simulink model "AutomatedValetParking"  (R2026a)
settings: Solver=VariableStepAuto  StopTime=inf  FixedStep=1e-3
PreLoadFcn:
  | costmap = VorlageCostmapErstellen();
  | routeData= load('routePlanSL.mat');
  | routePlan= routeData.routePlan;
  | startPose = routePlan.StartPose(1, :);
  | centerToFront = 1.4;
  | centerToRear = 1.4;
  | helperCreateBus;
StopFcn:
  | clear helperSLVisualizePath
values from neighbouring files (symbols this model uses):
  lr = vehDims.RearOverhang  + (vehDims.Wheelbase / 2)    [Initialisierung.m]
undefined symbols (not defined in the file or in its folder): DiscIntNeverNeededParam
libraries: drivingvehiclecontroller x2, drivinglib x2, simulink_extras x2, autolibshared x1
CloseFcn:
  | clear plannerConfigBus ...
  | speedConfigBus ...
  | startPose ...
  | costmap ...
  | routeData ...
  | routePlan ...
  | centerToFront ...
  | centerToRear;
settings Model: Creator=The MathWorks, Inc.  LastModifiedBy=moritzhumberg
settings SolverCC: DecoupledContinuousIntegration=on  MinimalZcImpactIntegration=on
settings DebuggingCC: PregeneratedLibrarySubsystemCodeDiagnostic=none
settings RTWCC: GenCodeOnly=on  PackageGeneratedCodeAndArtifacts=on

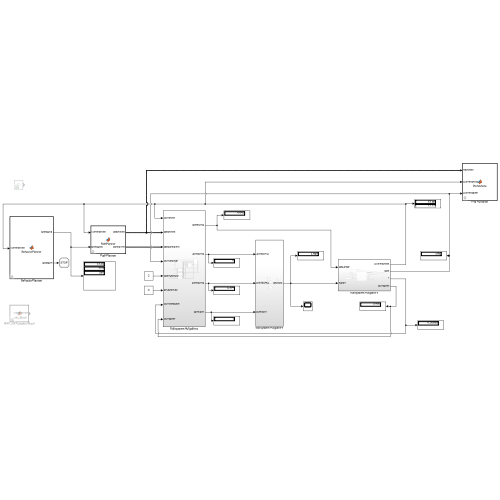
[thumbnail: Simulink's stored preview of the top-level diagram]
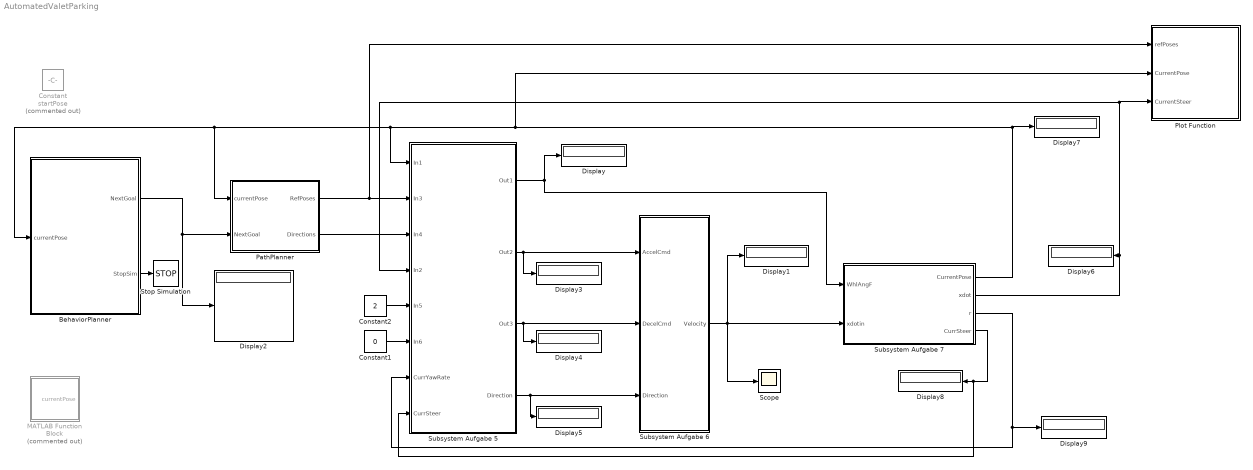
== system AutomatedValetParking ==
  BehaviorPlanner : MATLAB Function  TreatAsAtomicUnit=on  mask{routePlan=routePlan}
      mask init:
      | routePlanStruct = table2struct(routePlan);
  Constant : Constant  Commented=on  Value=startPose
  Constant1 : Constant  Value=0
  Constant2 : Constant  Value=2
  Display{,1..9} (10 alike) : Display
  MATLAB Function Block : MATLAB Function  Commented=on  TreatAsAtomicUnit=on
  PathPlanner : MATLAB Function  TreatAsAtomicUnit=on  mask{costmap=costmap}
      mask init:
      | varagout        = helperSLCreateUtilityStruct(costmap);
      |       vehicleDimsStruct = varagout{1};
      |       costmapStruct   = varagout{2};
  Plot Function : MATLAB Function  TreatAsAtomicUnit=on  mask{Costmap=costmap}
      mask init:
      | varagout        = helperSLCreateUtilityStruct(Costmap);
      |     vehicleDimsStruct = varagout{1};
      |     costmapStruct   = varagout{2};
  Scope : Scope
      settings: ActiveDisplayYMinimum=-1  ActiveDisplayYMaximum=1
  Stop Simulation : Stop
  Subsystem Aufgabe 5 : Subsystem
  Subsystem Aufgabe 6 : Subsystem
  Subsystem Aufgabe 7 : Subsystem
  wires:
  BehaviorPlanner/1(NextGoal) -> Display2/1, PathPlanner/2(NextGoal)
  PathPlanner/2(Directions) -> Subsystem Aufgabe 5/3(In4)
  PathPlanner/1(RefPoses) -> Plot Function/1(refPoses), Subsystem Aufgabe 5/2(In3)
  Constant2/1 -> Subsystem Aufgabe 5/5(In5)
  Subsystem Aufgabe 5/1(Out1) -> Subsystem Aufgabe 7/1(WhlAngF), Display/1
  Subsystem Aufgabe 6/1(Velocity) -> Scope/1, Subsystem Aufgabe 7/2(xdotin), Display1/1
  Subsystem Aufgabe 5/4(Direction) -> Display5/1, Subsystem Aufgabe 6/3(Direction)
  Subsystem Aufgabe 5/2(Out2) -> Display3/1, Subsystem Aufgabe 6/1(AccelCmd)
  Subsystem Aufgabe 5/3(Out3) -> Display4/1, Subsystem Aufgabe 6/2(DecelCmd)
  Subsystem Aufgabe 7/1(CurrentPose) -> Plot Function/2(CurrentPose), BehaviorPlanner/1(currentPose), PathPlanner/1(currentPose), Subsystem Aufgabe 5/1(In1), Display7/1
  Subsystem Aufgabe 7/2(xdot) -> Display6/1, Subsystem Aufgabe 5/4(In2), Plot Function/3(CurrentSteer)
  Subsystem Aufgabe 7/4(CurrSteer) -> Subsystem Aufgabe 5/8(CurrSteer), Display8/1
  Subsystem Aufgabe 7/3(r) -> Subsystem Aufgabe 5/7(CurrYawRate), Display9/1
  Constant1/1 -> Subsystem Aufgabe 5/6(In6)
  BehaviorPlanner/2(StopSim) -> Stop Simulation/1

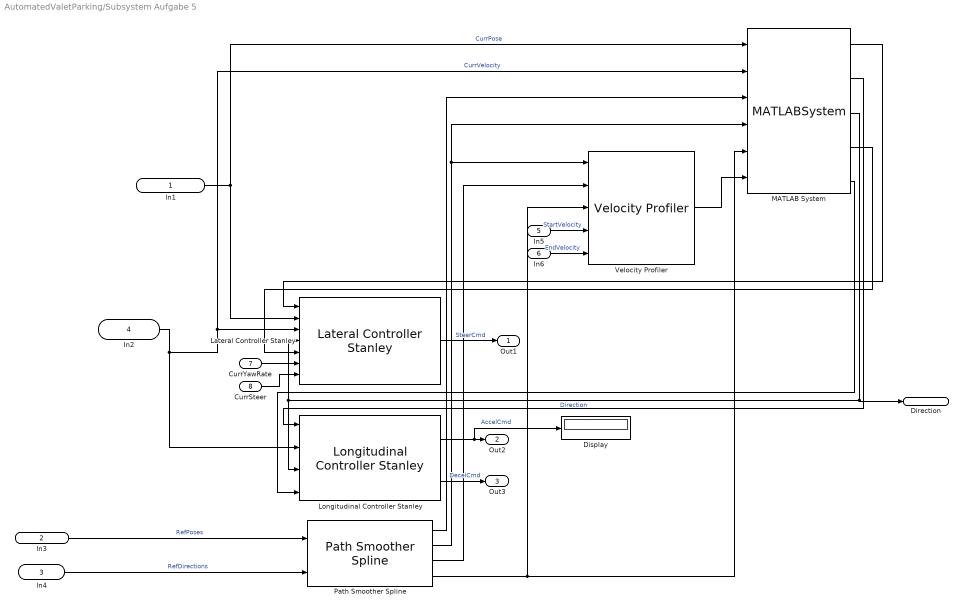
== system AutomatedValetParking/Subsystem Aufgabe 5 ==
  In1 : Inport
  In3 : Inport  Port=2
  In4 : Inport  Port=3
  In2 : Inport  Port=4
  In5 : Inport  Port=5
  In6 : Inport  Port=6
  CurrYawRate : Inport  Port=7
  CurrSteer : Inport  Port=8
  Display : Display
  Lateral Controller Stanley : drivingvehiclecontroller/Lateral Controller Stanley  ModelType=Dynamic bicycle model  PositionGainF=2.5  PositionGainR=2.5  YawRateGain=0.2  DelayGain=0.2  VehicleMass=1575  Lf=1.2  Lr=1.6  TireStiffness=19000  Wheelbase=2.8  MaxSteeringAngle=35
  Longitudinal Controller Stanley : drivingvehiclecontroller/Longitudinal Controller Stanley  Kp=2.5  Ki=1  SampleTime=0.1  MaxAcceleration=2  MaxDeceleration=4
  MATLAB System : MATLABSystem  System=HelperPathAnalyzer  Wheelbase=2.8  HasResetOutput=on  SimulateUsing=Interpreted execution
      mask Type: HelperPathAnalyzer
  Path Smoother Spline : drivinglib/Path Smoother Spline  NumSmoothPoses=100  MinSeparation=1e-3  SampleTime=0.1  ShowOptionalOutports=on  SimulateUsing=Interpreted execution
  Velocity Profiler : drivinglib/Velocity Profiler  MaxLongitudinalAccel=2  MaxLongitudinalDecel=4  MaxSpeed=10  MaxLongitudinalJerk=1  MaxLateralAccel=2  ShowOptionalOutport=off  SampleTime=-1  SimulateUsing=Code generation
  Out1 : Outport
  Out2 : Outport  Port=2
  Out3 : Outport  Port=3
  Direction : Outport  Port=4
  wires:
  In1/1 -> MATLAB System/1, Lateral Controller Stanley/2  "CurrPose"
  In2/1 -> Longitudinal Controller Stanley/2, MATLAB System/2, Lateral Controller Stanley/3  "CurrVelocity"
  In3/1 -> Path Smoother Spline/1  "RefPoses"
  Lateral Controller Stanley/1 -> Out1/1  "SteerCmd"
  Longitudinal Controller Stanley/1 -> Display/1, Out2/1  "AccelCmd"
  Longitudinal Controller Stanley/2 -> Out3/1  "DecelCmd"
  In5/1 -> Velocity Profiler/4  "StartVelocity"
  In6/1 -> Velocity Profiler/5  "EndVelocity"
  In4/1 -> Path Smoother Spline/2  "RefDirections"
  MATLAB System/3 -> Direction/1, Lateral Controller Stanley/4, Longitudinal Controller Stanley/3  "Direction"
  MATLAB System/1 -> Lateral Controller Stanley/1
  MATLAB System/2 -> Longitudinal Controller Stanley/1
  MATLAB System/5 -> Longitudinal Controller Stanley/4
  Path Smoother Spline/4 -> MATLAB System/5, Velocity Profiler/3
  Velocity Profiler/1 -> MATLAB System/6
  Path Smoother Spline/3 -> Velocity Profiler/2
  Path Smoother Spline/2 -> MATLAB System/4, Velocity Profiler/1
  Path Smoother Spline/1 -> MATLAB System/3
  MATLAB System/4 -> Lateral Controller Stanley/5
  CurrYawRate/1 -> Lateral Controller Stanley/6
  CurrSteer/1 -> Lateral Controller Stanley/7

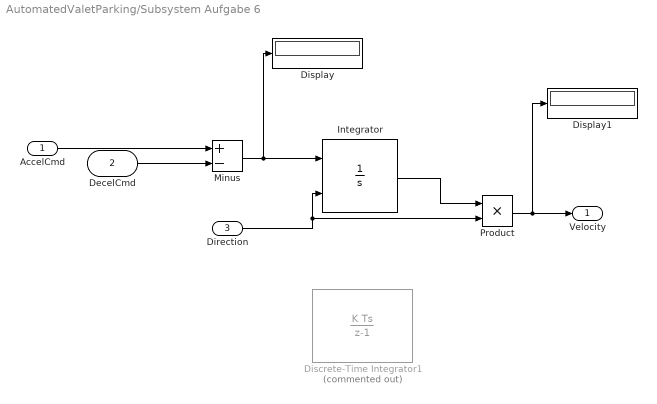
== system AutomatedValetParking/Subsystem Aufgabe 6 ==
  AccelCmd : Inport
  DecelCmd : Inport  Port=2
  Direction : Inport  Port=3
  Discrete-Time Integrator1 : DiscreteIntegrator  Commented=on  ExternalReset=either  InitialCondition=2  SampleTime=0.1  LimitOutput=on  LowerSaturationLimit=0  ICPrevOutput=DiscIntNeverNeededParam  ICPrevScaledInput=DiscIntNeverNeededParam
  Display : Display
  Display1 : Display
  Integrator : Integrator  ExternalReset=either  LimitOutput=on  LowerSaturationLimit=0
  Minus : Sum  Inputs=+-
  Product : Product
  Velocity : Outport
  wires:
  Minus/1 -> Integrator/1, Display/1
  DecelCmd/1 -> Minus/2
  AccelCmd/1 -> Minus/1
  Product/1 -> Velocity/1, Display1/1
  Direction/1 -> Integrator/2, Product/2
  Integrator/1 -> Product/1

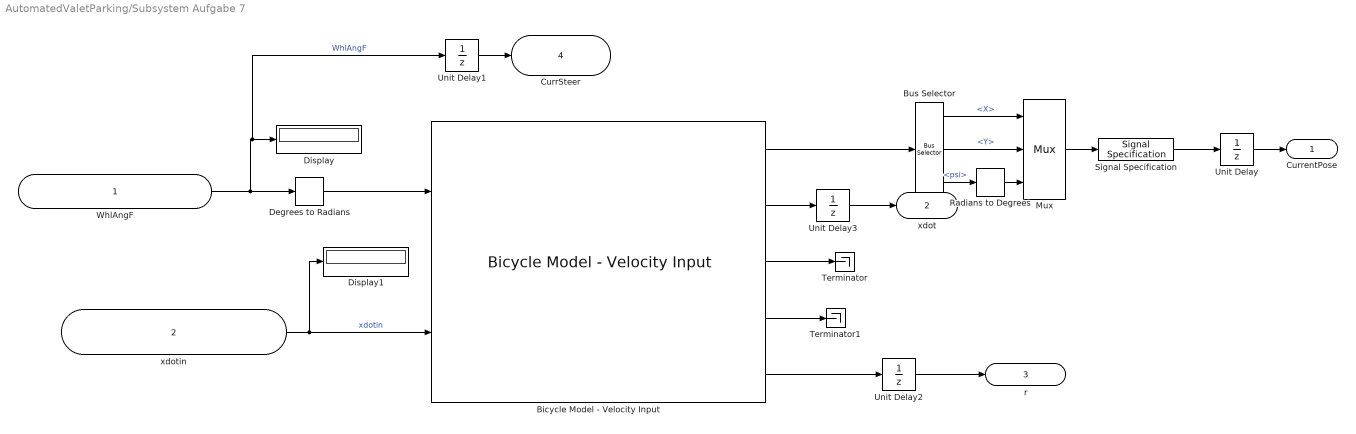
== system AutomatedValetParking/Subsystem Aufgabe 7 ==
  WhlAngF : Inport
  xdotin : Inport  Port=2
  Bicycle Model - Velocity Input : autolibshared/Bicycle Model - Velocity Input  trackMode=Single (bicycle)  inputMode=External longitudinal velocity  frontSteerMode=on  rearSteerMode=off  windMode=off  muMode=off  extFMode=off  extMMode=off  aMode=3  NF=2  NR=2  m=2000  a=lf  b=lr  h=0.35  X_o=startPose(1)  xdot_o=0  CalphaMode=Constant  sigmaMode=on  w=[1.4,1.4]  Cy_f=12e3  Cy_r=11e3  sigma_f=.1  sigma_r=.1  alpha_f_brk=[-.1 .1]  Cy_f_data=[-9e3 9e3]  alpha_r_brk=[-.1 .1]  Cy_r_data=[-9e3 9e3]  Y_o=startPose(2)  ydot_o=0  Izz=4000  psi_o=startPose(3)  r_o=0  Af=2  Cd=.3  Cl=.1  Cpm=.1  beta_w=[0 0.01:0.01:0.3]  Cs=[0 0.01:0.01:0.3]  Cym=[0 1e-6:0.01:0.3]  Pabs=101325  Tair=273  g=9.81  mu=1  xdot_tol=.01  Fznom=5000  Fxtire_sat=1e6  Fytire_sat=1e6  longOff=0  latOff=0  vertOff=0
      settings: LibrarySourceBlock=drivingscenarioandsensors/Bicycle Model - Velocity Input
  Bus Selector : BusSelector  OutputSignals=InertFrm.Cg.Disp.X,InertFrm.Cg.Disp.Y,InertFrm.Cg.Ang.psi
  Degrees to Radians : simulink_extras/Transformations/Degrees to Radians
  Display : Display
  Display1 : Display
  Mux : Mux  Inputs=3
  Radians to Degrees : simulink_extras/Transformations/Radians to Degrees
  Signal Specification : SignalSpecification  Dimensions=[1 3]
  Terminator : Terminator
  Terminator1 : Terminator
  Unit Delay : UnitDelay  InitialCondition=startPose  SampleTime=0.1
  Unit Delay1 : UnitDelay  SampleTime=-1
  Unit Delay2 : UnitDelay  SampleTime=-1
  Unit Delay3 : UnitDelay  SampleTime=-1
  CurrentPose : Outport
  xdot : Outport  Port=2
  r : Outport  Port=3
  CurrSteer : Outport  Port=4
  wires:
  Bicycle Model - Velocity Input/5 -> Unit Delay2/1
  Bicycle Model - Velocity Input/2 -> Unit Delay3/1
  WhlAngF/1 -> Unit Delay1/1, Display/1, Degrees to Radians/1  "WhlAngF"
  xdotin/1 -> Display1/1, Bicycle Model - Velocity Input/2  "xdotin"
  Degrees to Radians/1 -> Bicycle Model - Velocity Input/1
  Bicycle Model - Velocity Input/1 -> Bus Selector/1
  Bus Selector/1 -> Mux/1  "<X>"
  Bus Selector/2 -> Mux/2  "<Y>"
  Bus Selector/3 -> Radians to Degrees/1  "<psi>"
  Mux/1 -> Signal Specification/1
  Unit Delay1/1 -> CurrSteer/1
  Bicycle Model - Velocity Input/3 -> Terminator/1
  Bicycle Model - Velocity Input/4 -> Terminator1/1
  Unit Delay/1 -> CurrentPose/1
  Signal Specification/1 -> Unit Delay/1
  Unit Delay2/1 -> r/1
  Unit Delay3/1 -> xdot/1
  Radians to Degrees/1 -> Mux/3

== matlab function AutomatedValetParking/BehaviorPlanner ==
  settings: updateMethod=DISCRETE  sampleTime=0.1
  data: routePlanStruct parameter; NextGoal output size=1 3; currentPose input size=1 3; StopSim output
%% BehaviorPlanner
% Dieser Block soll aus dem routePlan die entsprechende Zielpose sowie 
% Geschwindigkeiten entnehmen und an dem motionPlaning Block
% weitergeben. Weiterhin soll der Block die Einstellung für den 
% RRT*-Algorithmus entsprechend der aktuellen Fahrsituation ermittlen und
% dem PathPlanner übergeben.
% Schließlich soll der Block nach dem Erreichen der finalen Zielpose die
% Simulation beenden.

% ------------------------------------------------------------------------------------------------------------
function [NextGoal, StopSim] = BehaviorPlanner(routePlanStruct, currentPose)

StopSim = false;
persistent GoalIndex;

if isempty(GoalIndex)
GoalIndex = 1; % Startwert
end

numGoals = length(routePlanStruct);

NextGoal = routePlanStruct(GoalIndex).EndPose;

dist = norm(currentPose(1:2) - NextGoal(1:2));

Toleranz = 0.8;




%% Aufgabe 3
% Nach der Definition der Ein- und Ausgänge der Function muss die Maske des
% Matlab Function Blocks definiert werden. Eine Besonderheit besteht darin,
% dass der routePlan aus Matlab geladen wird. 
% Aus diesem Grund ist dies kein klassischer Eingang vom Matlab 
% Function Block. 
% Unter Rechtsklick auf dem Matlab Function Block > Masks > Edit Mask...
% ist Parameters & Dialog zu finden. Dort können die Parameter definiert
% werden, die beim Doppelklick auf den Matlab Function Block definiert
% werden sollen.
% Unter dem Punkt Code lässt sich eine Intialisierungs Function
% definieren. Dieser Code wird benötigt um den routePlan in das Format
% "struct" zu konvertieren. Dies hat den Grund, dass Matlab Function Blöcke
% das Format "table" nicht unterstützen. Aus diesem Grund ist im Mask
% Editor unter Code über den Befehl 'S = table2struct(T)' eine Konvertierung
% des routePlans in ein Struct nötig. Ein Struct ist ein Datenformat, der
% aus einem großen "Container" besteht, in dem mehrere Werte eingegliedert
% sind. So lässt sich eine geordnetere Datenstruktur bilden.
% Weitere Erläuterungen zur Mask befinden sich unter Kapitel 5.3 in den
% Praktikumsunterlagen Aufgabenstellung.

% -

% Wenn nur eine erste Zielpose ausgegeben werden soll, reicht die
% Implementierung des GoalIndexes und der einfache
% Befehl x = routePlanStruct(Index).EndPose
%                  |           |        |
%           Variablenname  Zeilennr.  Spalte
% Der GoalIndex ist in dieser Aufgabe nur eine Konstante, da lediglich die 
% erste Zielpose aufgerufen werden soll. 
% In den aufbauenden Aufgaben wird dies aber eine laufende Nummer, die
% nacheinander alle Zielposen aus dem dem RoutePlan aufruft.
% Dieser Schritt wird in folgenden Aufgaben aber in requestManeuver.m
% ausgelagert, da dies bei komplexeren Anwendungen Vorteile hat. Diese
% liegen beispielsweise bei einer besseren Übersichtlichkeit. Außerdem
% können diese ausgelagerten Skripte von verschiedenen Stellen (bsp. von 
% mehreren Matlab Function Blöcken) aufgerufen werden.

% --------------------------------------------------------------------------
%% Aufgabe 9
% Für die Lösung dieser Aufgabe muss die, bereits in Aufgabe 3
% angesprochene, Variable GoalIndex zu einer laufenden Nummer erweitert
% werden. Dazu sind auch wieder persistente Variablen wie in Aufgabe 5
% nötig.
% Weiterhin ist eine if-Bedingung nötig, die die nächste Zielpose aus dem
% routePlan entnimmt und anschließen den GoalIndex um einen Zähler erhöht, 
% wenn das Ego-Fahrzeug die aktuelle Zielpose erreicht. Dies ist über die 
% Beobachtung der Distanz zur Zielpose realisierbar.

if dist < Toleranz
    if GoalIndex < numGoals % Nicht bei Index 6 (Letzter Index im Array routeplanstruct
        GoalIndex = GoalIndex + 1;
        NextGoal = routePlanStruct(GoalIndex).EndPose;

% -------------------------------------------------------------------------- 
%% Aufgabe 10
% Bei dieser Aufgabe kann auf dem Code aus Aufgabe 9 aufgebaut werden. Für
% die Lösung muss lediglich ein weiterer Ausgang mit einer Variable in den 
% "Matlab Function"-Block ergänzt werden, die bei Erreichung der finalen
% Zielpose den "Stop Simulation"-Block aktiviert. Dazu ist zu Beginn des
% Codes eine Initialisierung der Variable nötig und eine weitere
% if-Bedingung, die ausgelöst wird, wenn die Distanz zu der finalen
% Zielpose einen definierten Wert unterschreitet.

    else %letztes Ziel erreicht
        StopSim = true;
    end
end

% ------------------------------------------------------------------------------------------------------------  
%% Aufgabe 11
% Bei dieser Aufgabe können Sie die vorher genutzte Logik in das Skript
% "requestManeuver.m" überführen. Damit können Sie auch die Variable
% aus diesem Code löschen und nur noch in dem ausgelagerten Skript
% einsetzen.
% Für den Aufruf eines Matlab Skriptes aus dem Matlab Function Block muss
% der Name der Function zusammen mit den Ein- und Ausgabe-Variablen 
% aufegrufen werden.
% Beispiel: 
%           function im Matlab Skript
%               function z = Addition(x,y)
%           
%                   z = x + y;
%
%               end
%
%           Aufruf der function im Matlab Function Block: 
%               z = Addition(x,y);

% ------------------------------------------------------------------------------------------------------------  
%% Aufgabe 12
% Für diese Aufgabe muss die Function y = speedSettings(u) in der Datei
% "requestManeuver.m" eingeführt und dem BehaviorPlanner übergeben werden.
% --
% Da ein Struct mehrere Werte umfasst, ist dieser nicht auf "normalen"
% Wege einem anderen Simulink-Block übermittelbar. Darum findet hier der
% Typ "Bus" Anwendung. Wie dieser eingesetzt wird, ist in der
% Aufgabenstellung unter Property Inspector beschrieben. Wichtig ist dabei,
% dass Bezeichnungen aus der Helper-Datei "helperCreateBus.m" sich
% hier in den Variablennamen wiederfinden und allgemein auch die Formate
% sowie Datentypen übereinstimmen. Außerdem muss im Property Inspector der
% Busname manuell eingetippt werden. Dabei ist zu beachten, dass die Form
% "Bus: Busname" lautet.

% -----------------------------------------------------------------------------------------------------------
%% Aufgabe 13
% Bei dieser Aufgabe muss ähnlich wie in Aufgabe 12 vorgegangen werden. In
% der Datei "requestManeuver.m" muss die Function "y = plannerSettings(u)"
% nochmals erweitert werden, sodass je nach Fahrmanöver die Einstellungen
% für den RRT*-Algorithmus bestimmt werden. Diese müssen anschließend über
% den Bus namens "plannerConfigBus" dem PathPlanner übergeben und dort von
% dem Befehl "planner = pathPlannerRRT(costmap,Name,Value);"
% entgegengenommen werden.

end

== matlab function AutomatedValetParking/MATLAB Function Block ==
  data: currentPose output double size=[1 3]
function currentPose = Funki_Block()
    currentPose = [4, 12, 0];  % [X, Y, Theta]
end

== matlab function AutomatedValetParking/PathPlanner ==
  settings: updateMethod=DISCRETE  sampleTime=0.1
  data: currentPose input size=1 3; NextGoal input size=[1 3]; RefPoses output size=100 3; Directions output size=100 1; costmapStruct parameter; vehicleDimsStruct parameter
%% PathPlanner
% Dieses Skript soll die nächste Zielpose und die aktuelle Pose
% entgegennehmen. Mithilfe des RRT*-Algorithmus soll die entsprechende Route
% bestimmt werden. Der PathPlanner-Block soll dann die refPoses und die
% direction ausgeben.
% Auch hier sind die Kommentare den einzelnen Aufgaben zugewiesen.
%--------------------------------------------------------------------------
function [RefPoses, Directions]  = PathPlanner(currentPose, NextGoal, costmapStruct, vehicleDimsStruct)   
%% Aufgabe 4 
    % Über die Maske muss die Costmap geladen werden. Außerdem muss in der
    % Callback Function die helper-Datei helperSLCreateUtilityStruct.m
    % aufgerufen werden. Hier lässt sich der vehicleDimsStruct und der
    % costmapStruct ermitteln.
    % function initialization()
    % 
    %       varagout        = helperSLCreateUtilityStruct(Costmap);
    %       vehicleDimsStruct = varagout{1};
    %       costmapStruct   = varagout{2};
    %
    % end

    % Hinweis: Die Eingänge costmapStruct und vehicleDimsStruct dürfen im
    % Property Inspector nicht als "tunable" deklariert sein.
    % Die Einstellungen für "Size" müssen für die Werte currentPose, 
    % RefPoses und Directions müssen im Property Inspector geändert werden.
    % currentPose: [1 3], RefPoses: [100 3] Directions: [100 1]
% ---------------------------------–-----------------–-----------------–-----------------–
%% Aufgabe 5   
    % Zu Beginn müssen einige Variablen als persistent definiert werden. Dies
    % hat den Zweck, dass die Variablen lokal im Skript gespeichert werden.
    % Ansonsten werden diese immer wieder zurückgesetzt.
    % Zu der Definition einer persistenten Variable gehört auch die Bestimmung
    % mit welchem Wert die Variable initiiert werden soll. Dazu wird
    % üblicherweise die if-Bedingung "if isempty" verwendet. Diese Bedingung
    % überprüft, ob der Variable schon ein Wert zugewiesen ist. Falls dies
    % nicht der Fall ist, ist in der Bedingung zu definieren welcher Startwert
    % angewendet werden soll.
    % Für jede persistente Variable muss so eine "if isempty"-Bedingung 
    % durchlaufen werden. Optional ist auch eine if ~exist möglich.
    % Persistente Variablen können nicht direkt von dem Matlab Function Block
    % ausgegeben werden. Daher muss immer folgender beispielhafter Ablauf
    % eingehalten werden:
    % 
    % function x_Ausgang = Beispielfunction()
    %
    % persistent x
    % if isempty x
    %   x = 0;
    % end
    %
    % //Code//
    %
    % x_Ausgang = x
    persistent nextGoal refPoses directions

    if isempty(nextGoal)
        nextGoal = [0 0 0];
    end

    if isempty(refPoses)
        refPoses = [0 0 0];
    end

    if isempty(directions)
        directions = 1;
    end

% ---------------------------------–-----------------–-----------------–-----------------–    
%% Aufgabe 4    
    % Für die Erkennung von Kollisionen müssen die Dimensionen vom Fahrzeug
    % parametrisiert werden. Diese umfassen die Werte, die schon bei dem Befehl 
    % 'vehicleCostmap' zur Erstellung der Costmap in Aufgabe 1 angesprochen wurden.
    % Mit den Dimensionen kann nun die Variable 'vehicleDims' bestimmt werden.
    % Dies ist durch den Befehl 'vdims = vehicleDimensions(l,w,h)' möglich.
    % Dieser Wert wird von dem 'inflationCollisionChecker' benötigt.
    % Der inflationCollisionChecker vergrößert die sich auf der Costmap
    % befindenden Hindernisse. Somit wird automatisch ein bestimmter
    % Sicherheitsabstand implementiert. Für den 'inflationCollisionChecker'
    % soll die Variable "vehicleDims" für die Fahrzeugdimensionen und der Wert
    % 4 für die Variable "numCircles" verwendet werden.

    vehicleDims = vehicleDimensions( ...
        vehicleDimsStruct.Length, ...
        vehicleDimsStruct.Width, ...
        vehicleDimsStruct.Height);
        % 'Wheelbase',          vehicleDimsStruct.Wheelbase, ...
        % "RearOverhang", vehicleDimsStruct.RearOverhang, ...
        % "FrontOverhang", vehicleDimsStruct.FrontOverhang, ...
        % "WorldUnits", vehicleDimsStruct.WorldUnits);

    % vehicleDims = vehicleDimensions( ...
    % vehicleDimsStruct.Length, ...
    % vehicleDimsStruct.Width, ...
    % vehicleDimsStruct.Height, ...
    % 'Wheelbase',          vehicleDimsStruct.Wheelbase, ...
    % 'RearOverhang',       vehicleDimsStruct.RearOverhang, ...
    % 'WorldUnits',         char(vehicleDimsStruct.WorldUnits));
    
    CollisionChecker = inflationCollisionChecker(vehicleDims, 4);
    
    % Nun wird eine neue Costmap erstellt. Diese bildet sich erneut durch den
    % Befehl 'costmap = vehicleCostmap(C)' und die Werte im costmapStruct. 
    % Die Werte umfassen:
    % Costs, FreeThreshold, OccupiedThreshold, CellSize und CollisionChecker
    % Zudem wird hier auch eine CellSize und der inflationCollisionChecker beachtet.
    % Der Befehl lautet 'costmap = vehicleCostmap(costmapStruct.Costs, ...
    %                                   'FreeThreshold',costmapStruct.FreeThreshold, ...
    %                                   'OccupiedThreshold', costmapStruct.OccupiedThreshold, ...
    %                                   'MapLocation', costmapStruct.MapExtent([1, 3]), ...
    %                                   'CellSize', costmapStruct.CellSize, ...
    %                                   'CollisionChecker', CollisionChecker);

    Costmap = vehicleCostmap(costmapStruct.Costs, ...
                             'FreeThreshold',costmapStruct.FreeThreshold, ...
                             'OccupiedThreshold', costmapStruct.OccupiedThreshold, ...
                             'MapLocation', costmapStruct.MapExtent([1, 3]), ...
                             'CellSize', costmapStruct.CellSize, ...
                             'CollisionChecker', CollisionChecker);
   
    % Mit der neu erstellten costmap kann nun der RRT*-Algorithmus arbeiten. Der
    % RRT*-Algorithmus wird über den Befehl 
    % 'planner = pathPlannerRRT(costmap,Name,Value);' aufgerufen. Der
    % RRT*-Algorithmus muss noch so eingestellt werden, dass er möglichst
    % effizient und sicher arbeitet. (ConnectionStistance, MinIterations,
    % GoalDistance, MinTurningRadius). 
    % Im Rahmen von Aufgabe 4 reicht es ist es diese Werte frei zu wählen. 
    % Dafür bietet sich beispielsweise für ConnectionDistance ein 
    % Wert von 10 an, für MinIterations 2000, für GoalTolerance [0.5 0.5 5] 
    % und für MinTurningRadius 10. 

    planner = pathPlannerRRT(Costmap, ...
        'ConnectionDistance', 5, ...
        'MinIterations',      4000, ...
        'GoalTolerance',      [0.5 0.5 5], ...
        'MinTurningRadius',   5);

 %----
 %% Aufgabe 13
    % Da sich die passende Einstellung von Fahrsituation zu Fahrsituation
    % ändert, soll die passende Einstellung des RRT*-Algorithmus von der 
    % function requestManeuver bestimmt werden und über den 
    % plannerConfig-Bus (helperCreateBus.m) dem PathPlanner übergeben 
    % werden. Daher soll in diesem Abschnitt der Befehl 
    % 'planner = pathPlannerRRT(costmap,Name,Value);'nochmal überarbeitet
    % werden. 

% ---------------------------------–-----------------–-----------------–-----------------–    
%% Aufgabe 4
% refPoses = plan(planner, currentPose, NextGoal);
% 
% [RefPoses, Directions] = interpolate(refPoses);
    % Mit dem Befehl 'planner = pathPlannerRRT(costmap,Name,Value);'
    % erfolgt lediglich die Parametrierung des RRT-Algorithmus. Der
    % tatsächliche Einsatz erfolgt erst jetzt. 
    % Der Befehl 'refPath = plan(planner,startPose,goalPose);' ermittelt
    % den Pfad. Der Befehl '[RefPoses, Directions] = interpolate(refPath);
    % ermittelt aus dem Pfad die einzelnen Posen und die Fahrtrichtung. Für
    % die Lösung der Aufgabe 4 soll lediglich die Funktion des 
    % RRT*-Algorithmus und die Ermittlung der RefPoses sowie der
    % Fahrtrichtung nachgewiesen werden. In Aufgabe 5 wird der Code nochmal
    % angepasst, sodass die RefPose und die Fahrtrichtung nur neu ermittelt
    % werden, wenn auch wirklich eine neue Zielpose vorliegt.
    % 
 %----
 %% Aufgabe 5
    % Die refPoses und Directiosn sollen nur neu berechnet werden, wenn 
    % auch wirklich eine neue Route benötigt wird. 
    % Dies ist der Fall, wenn die aktuelle Pose auf dem sich das 
    % Ego-Fahrzeug befindet mit der letzten ZielPose übereinstimmt.
    % Eine entsprechende if ~isequal - else - Bedingung soll dies überprüfen.
    % Bei jedem Durchlauf dieses Skripts soll eine Speicherung der 
    % aktuellen Zielpose erfolgen. Falls die Zielpose beim nächsten
    % Durchlauf mit der, des letzen Durchlaufes übereinstimmt, soll nichts
    % passieren. Sobald aber eine neue Zielpose vorhanden ist, soll der 
    % RRT-Algorithmus aktiv werden und neue RefPoses sowie Directions 
    % (Angabe der Fahrtrichtung) erzeugen. Dies soll mit dem Befehl
    % 'refPath = plan(planner,startPose,goalPose);' und
    % '[RefPoses, Directions] = interpolate(refPath);' erfolgen.
    % Sobald die Variablen RefPoses und Directions bestimmt werden ist die
    % Aufgabe dieses Skripts erledigt.

    if ~isequal(nextGoal, NextGoal)
        refPath = plan(planner, currentPose, NextGoal);
        [RefPoses, Directions] = interpolate(refPath);

        nextGoal = NextGoal;
        refPoses = RefPoses;
        directions = Directions;

    else
        RefPoses = refPoses;
        Directions = directions;

    end

end

== matlab function AutomatedValetParking/Plot Function ==
  data: refPoses input; CurrentPose input; costmapStruct parameter; vehicleDimsStruct parameter; CurrentSteer input
function PlotVehicle(refPoses, CurrentPose, costmapStruct, vehicleDimsStruct, CurrentSteer)

coder.extrinsic('helperSLVisualizePath')

helperSLVisualizePath(CurrentPose, CurrentSteer, refPoses, costmapStruct, vehicleDimsStruct);
